simulink model "roll_and_yaw_damper"  (R2018b)
settings: Solver=VariableStepAuto  StartTime=0.0  StopTime=100  RelTol=1e-3
libraries: cstblocks x1
settings Model: Creator=FARYAL  LastModifiedBy=FARYAL

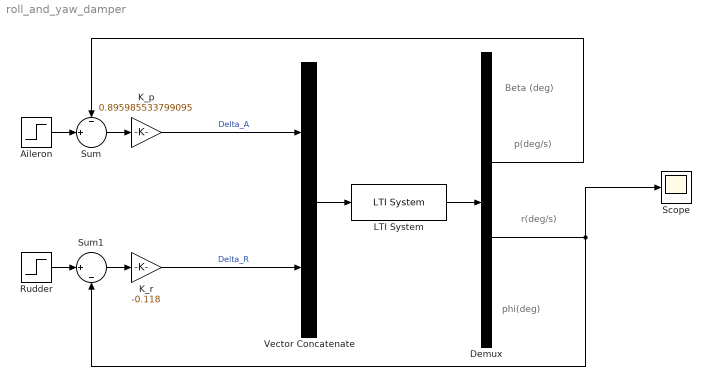
== system roll_and_yaw_damper ==
  note: Beta (deg)
  note: p(deg/s)
  note: phi(deg)
  note: r(deg/s)
  Aileron : Step  SampleTime=0
  Demux : Demux
  K_p : Gain  Gain=0.895985533799095
  "K_r " : Gain  Gain=-0.118
  LTI System : cstblocks/LTI System  sys=System  IC=[]
  Rudder : Step  After=0  SampleTime=0
  Scope : Scope
  Sum : Sum  Inputs=-|+||
  Sum1 : Sum  Inputs=||+|-
  Vector Concatenate : Concatenate
  wires:
  Aileron/1 -> Sum/2
  LTI System/1 -> Demux/1
  "K_r "/1 -> Vector Concatenate/2  "Delta_R"
  Sum1/1 -> "K_r "/1
  Demux/2 -> Sum/1
  Rudder/1 -> Sum1/1
  Vector Concatenate/1 -> LTI System/1
  Sum/1 -> K_p/1
  K_p/1 -> Vector Concatenate/1  "Delta_A"
  Demux/3 -> Scope/1, Sum1/2
